simulink model "PI_VC_vs_UPI_CC_3ph_4w_v2023b"  (R2023b)
settings: Solver=FixedStepDiscrete  StartTime=0.0  StopTime=14  FixedStep=Ts_Power  MaxStep=1e-4  RelTol=1e-3
InitFcn:
  | run PI_VC_vs_UPI_CC_ini;
values from neighbouring files (symbols this model uses):
  C = 4e-6    (= 4e-06)    [PI_OL_vs_PI_CC_ini.m]    (also in PI_VC_vs_UPI_CC_ini.m)
  C_2 = 4e-6    (= 4e-06)    [PI_OL_vs_PI_CC_ini.m]    (also in PI_VC_vs_UPI_CC_ini.m)
  K_i_pll = 1.8/0.00251    (= 717.131474104)    [PI_OL_vs_PI_CC_ini.m]    (also in PI_VC_vs_UPI_CC_ini.m)
  K_p_pll = 1.8    [PI_OL_vs_PI_CC_ini.m]    (also in PI_VC_vs_UPI_CC_ini.m)
  Kp_i = 1*(L_t2 + L_s2)/tau_i    (= 2.5)    [PI_OL_vs_PI_CC_ini.m]    (also in PI_VC_vs_UPI_CC_ini.m)
  Kr_i = 2*(R_t2 + R_s2)/tau_i    (= 157.079632679)    [PI_OL_vs_PI_CC_ini.m]    (also in PI_VC_vs_UPI_CC_ini.m)
  L_line_12_13 = X_line_12_13/(2*pi*50)    (= 0.000798957814321)    [PI_OL_vs_PI_CC_ini.m]    (also in PI_VC_vs_UPI_CC_ini.m)
  L_line_13_14 = X_line_13_14/(2*pi*50)    (= 0.000200535228296)    [PI_OL_vs_PI_CC_ini.m]    (also in PI_VC_vs_UPI_CC_ini.m)
  L_n = L_t2 + L_s2    (= 0.0025)    [PI_OL_vs_PI_CC_ini.m]    (also in PI_VC_vs_UPI_CC_ini.m)
  L_s = 1.25e-3    (= 0.00125)    [PI_OL_vs_PI_CC_ini.m]    (also in PI_VC_vs_UPI_CC_ini.m)
  L_s2 = 1.25e-3    (= 0.00125)    [PI_OL_vs_PI_CC_ini.m]    (also in PI_VC_vs_UPI_CC_ini.m)
  L_t = 1.25e-3    (= 0.00125)    [PI_OL_vs_PI_CC_ini.m]    (also in PI_VC_vs_UPI_CC_ini.m)
  L_t2 = 1.25e-3    (= 0.00125)    [PI_OL_vs_PI_CC_ini.m]    (also in PI_VC_vs_UPI_CC_ini.m)
  omega = 2*pi*f    (= 314.159265359)    [PI_OL_vs_PI_CC_ini.m]    (also in PI_VC_vs_UPI_CC_ini.m)
  params_pi_cc = [S_b,U_b,K_p,T_p,K_q,T_q,X,R]    [PI_OL_vs_PI_CC_ini.m]    (also in PI_VC_vs_UPI_CC_ini.m)
  params_pi_vc = [S_b,U_b,K_p,T_p,K_q,T_q,Xv,Rv]    [PI_OL_vs_PI_CC_ini.m]    (also in PI_VC_vs_UPI_CC_ini.m)
  params_vc_cc = [R_t;L_t;R_s;L_s;K_pi;K_ii;C;K_pv;K_iv]    [PI_OL_vs_PI_CC_ini.m]    (also in PI_VC_vs_UPI_CC_ini.m)
  R_d = 10    [PI_OL_vs_PI_CC_ini.m]    (also in PI_VC_vs_UPI_CC_ini.m)
  R_d2 = 10    [PI_OL_vs_PI_CC_ini.m]    (also in PI_VC_vs_UPI_CC_ini.m)
  R_line_12_13 = (0.06)*Length    (= 0.24)    [PI_OL_vs_PI_CC_ini.m]    (also in PI_VC_vs_UPI_CC_ini.m)
  R_line_13_14 = (0.025)*Length    (= 0.1)    [PI_OL_vs_PI_CC_ini.m]    (also in PI_VC_vs_UPI_CC_ini.m)
  R_n = L_n*omega/10    (= 0.0785398163397)    [PI_OL_vs_PI_CC_ini.m]    (also in PI_VC_vs_UPI_CC_ini.m)
  R_s = L_s*omega/10    (= 0.0392699081699)    [PI_OL_vs_PI_CC_ini.m]    (also in PI_VC_vs_UPI_CC_ini.m)
  R_s2 = L_s*omega/10    (= 0.0392699081699)    [PI_OL_vs_PI_CC_ini.m]    (also in PI_VC_vs_UPI_CC_ini.m)
  R_t = L_t*omega/10    (= 0.0392699081699)    [PI_OL_vs_PI_CC_ini.m]    (also in PI_VC_vs_UPI_CC_ini.m)
  R_t2 = L_t*omega/10    (= 0.0392699081699)    [PI_OL_vs_PI_CC_ini.m]    (also in PI_VC_vs_UPI_CC_ini.m)
  S_b = 20e3    (= 20000)    [PI_OL_vs_PI_CC_ini.m]    (also in PI_VC_vs_UPI_CC_ini.m)
  Ts_Control = 50e-6    (= 5e-05)    [PI_OL_vs_PI_CC_ini.m]    (also in PI_VC_vs_UPI_CC_ini.m)
  Ts_Power = 50e-6    (= 5e-05)    [PI_OL_vs_PI_CC_ini.m]    (also in PI_VC_vs_UPI_CC_ini.m)
  v_dc = 800    [PI_OL_vs_PI_CC_ini.m]    (also in PI_VC_vs_UPI_CC_ini.m)
undefined symbols (not defined in the file or in its folder): DiscIntNeverNeededParam, omega_ref
libraries: spsFirstOrderFilterLib x32, spsUniversalBridgeLib x10, spsThreePhaseSeriesRLCBranchLib x9, spsPowerLib x6, spsThreePhaseVIMeasurementLib x6, eeGeneralControl x5, spsSeriesRLCLoadLib x5, spsRMSLib x4, spsSeriesRLCBranchLib x4, spsPower3phInstantaneousLib x3, spsThreePhaseBreakerLib x3, spsDCVoltageSourceLib x2
(part 1 of 3)
settings Model: Creator=Manuel  LastModifiedBy=iberi
settings SolverCC: AlgebraicLoopSolver=TrustRegion
settings DataIOCC: ReturnWorkspaceOutputs=off
settings DebuggingCC: UnconnectedInputMsg=warning  UnconnectedOutputMsg=warning  UnconnectedLineMsg=warning  ArithmeticOperatorsInVariantConditions=warning
settings ModelReferenceCC: EnableRefExpFcnMdlSchedulingChecks=on
settings SFSimCC: SimUseLocalCustomCode=off  CustomCodeUndefinedFunction=UseInterfaceOnly
settings RTWCC: RTWUseLocalCustomCode=off  DLArmComputeVersion=19.05

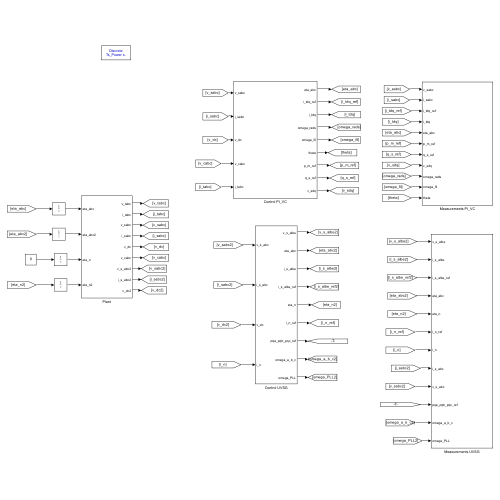
[thumbnail: Simulink's stored preview of the top-level diagram]
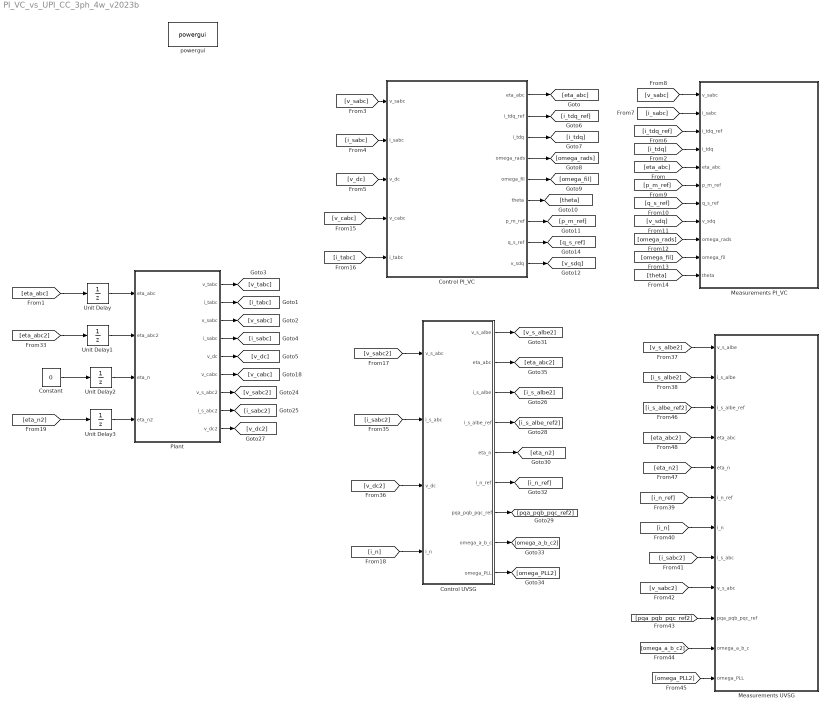
== system PI_VC_vs_UPI_CC_3ph_4w_v2023b ==
  Constant : Constant  Value=0
  Control PI_VC : Subsystem
  Control UVSG : Subsystem
  Measurements PI_VC : Subsystem
  Measurements UVSG : Subsystem
  Plant : Subsystem
  Unit Delay{,1..3} (4 alike) : UnitDelay  SampleTime=-1  HasFrameUpgradeWarning=on
  powergui : spspowerguiLib/powergui  Priority=1  SimulationMode=Discrete  SampleTime=Ts_Power  frequency=60  Iterations=50  frequencyindice=0  Pbase=100e6  ErrMax=1e-4  UnitsV=kV  UnitsW=MW  buscounter=0  FunctionMessages=off  echomessages=off  EnableUseOfTLC=off  CurrentSourceSwitches=off  DisableSnubberDevices=off  DisableRonSwitches=off  DisableVfSwitches=off  DisplayEquations=off  AutomaticDiscreteSolvers=off  SolverType=Tustin/Backward Euler (TBE)  Interpol=off  ExternalGateDelay=off  methode=off  Ts=100  x0status=blocks  SPID=on  SwTol=0  HookPort=off  NonlinearTolerance=1e-4  nMaxIteration=100  ContinueOnMaxIteration=off  RestoreLinks=warning  ResistiveCurrentMeasurement=off  Frange=[0:2:500]  Ylog=off  Xlog=on  ShowGrid=off  save=off  variable=ZData  structure=v_sabc  ZoomFFT=off  StartTime=4  cycles=5  DisplayStyle=2  fundamental=50  FreqAxis=off  MaxFrequency=10000  frequencyindicesteady=1  RmsSteady=1  display=off
  wires:
  [v_sabc] -> Control PI_VC/1(v_sabc)
  [i_sabc] -> Control PI_VC/2(i_sabc)
  [v_dc] -> Control PI_VC/3(v_dc)
  Control PI_VC/1(eta_abc) -> [eta_abc]
  Control PI_VC/2(i_tdq_ref) -> [i_tdq_ref]
  Control PI_VC/3(i_tdq) -> [i_tdq]
  Control PI_VC/4(omega_rads) -> [omega_rads]
  Control PI_VC/5(omega_fil) -> [omega_fil]
  Control PI_VC/6(theta) -> [theta]
  Control PI_VC/7(p_m_ref) -> [p_m_ref]
  Control PI_VC/8(q_s_ref) -> [q_s_ref]
  Control PI_VC/9(v_sdq) -> [v_sdq]
  [eta_abc] -> Measurements PI_VC/5(eta_abc)
  [i_tdq] -> Measurements PI_VC/4(i_tdq)
  [i_tdq_ref] -> Measurements PI_VC/3(i_tdq_ref)
  [i_sabc] -> Measurements PI_VC/2(i_sabc)
  [v_sabc] -> Measurements PI_VC/1(v_sabc)
  [p_m_ref] -> Measurements PI_VC/6(p_m_ref)
  [q_s_ref] -> Measurements PI_VC/7(q_s_ref)
  [v_sdq] -> Measurements PI_VC/8(v_sdq)
  [omega_rads] -> Measurements PI_VC/9(omega_rads)
  [omega_fil] -> Measurements PI_VC/10(omega_fil)
  [theta] -> Measurements PI_VC/11(theta)
  [v_cabc] -> Control PI_VC/4(v_cabc)
  [i_tabc] -> Control PI_VC/5(i_tabc)
  Plant/2(i_tabc) -> [i_tabc]
  Plant/6(v_cabc) -> [v_cabc]
  [eta_abc2] -> Unit Delay1/1
  [eta_abc] -> Unit Delay/1
  Plant/7(v_s_abc2) -> [v_sabc2]
  Plant/9(v_dc2) -> [v_dc2]
  Constant/1 -> Unit Delay2/1
  Unit Delay/1 -> Plant/1(eta_abc)
  Plant/5(v_dc) -> [v_dc]
  Unit Delay1/1 -> Plant/2(eta_abc2)
  Plant/8(i_s_abc2) -> [i_sabc2]
  Plant/3(v_sabc) -> [v_sabc]
  Plant/1(v_tabc) -> [v_tabc]
  Plant/4(i_sabc) -> [i_sabc]
  Unit Delay2/1 -> Plant/3(eta_n)
  [eta_n2] -> Unit Delay3/1
  Unit Delay3/1 -> Plant/4(eta_n2)
  Control UVSG/4(i_s_albe_ref) -> [i_s_albe_ref2]
  Control UVSG/5(eta_n) -> [eta_n2]
  [i_sabc2] -> Control UVSG/2(i_s_abc)
  [i_s_albe2] -> Measurements UVSG/2(i_s_albe)
  [v_s_albe2] -> Measurements UVSG/1(v_s_albe)
  [i_n] -> Measurements UVSG/7(i_n)
  [v_sabc2] -> Control UVSG/1(v_s_abc)
  [eta_abc2] -> Measurements UVSG/4(eta_abc)
  [i_s_albe_ref2] -> Measurements UVSG/3(i_s_albe_ref)
  [v_dc2] -> Control UVSG/3(v_dc)
  Control UVSG/9(omega_PLL) -> [omega_PLL2]
  Control UVSG/6(i_n_ref) -> [i_n_ref]
  [v_sabc2] -> Measurements UVSG/9(v_s_abc)
  [pqa_pqb_pqc_ref2] -> Measurements UVSG/10(pqa_pqb_pqc_ref)
  [omega_a_b_c2] -> Measurements UVSG/11(omega_a_b_c)
  Control UVSG/7(pqa_pqb_pqc_ref) -> [pqa_pqb_pqc_ref2]
  [i_sabc2] -> Measurements UVSG/8(i_s_abc)
  Control UVSG/8(omega_a_b_c) -> [omega_a_b_c2]
  [eta_n2] -> Measurements UVSG/5(eta_n)
  [omega_PLL2] -> Measurements UVSG/12(omega_PLL)
  [i_n] -> Control UVSG/4(i_n)
  [i_n_ref] -> Measurements UVSG/6(i_n_ref)
  Control UVSG/2(eta_abc) -> [eta_abc2]
  Control UVSG/3(i_s_albe) -> [i_s_albe2]
  Control UVSG/1(v_s_albe) -> [v_s_albe2]

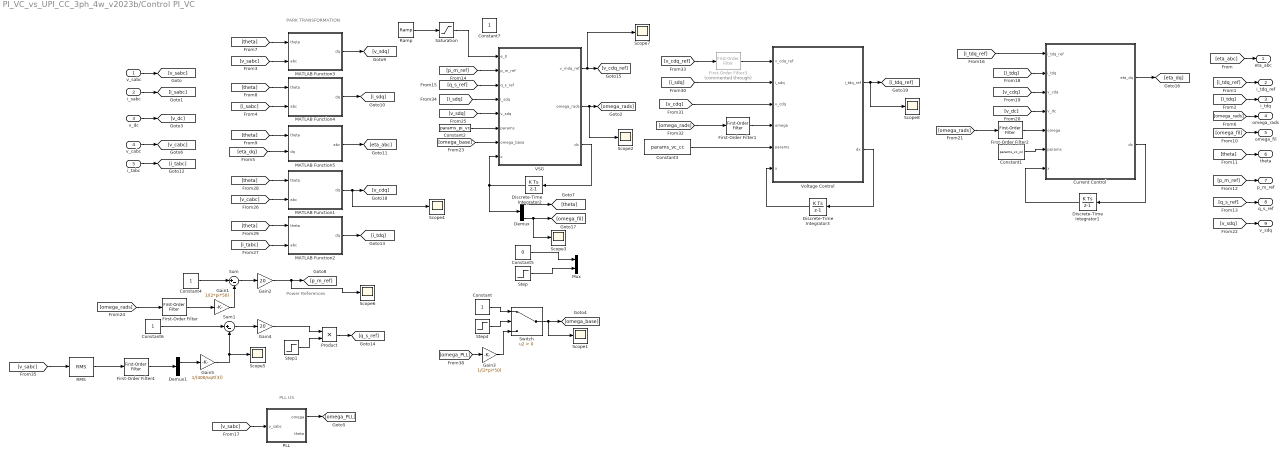
== system PI_VC_vs_UPI_CC_3ph_4w_v2023b/Control PI_VC ==
  note: PARK TRANSFORMATION
  note: Power References
  note: PLL US
  v_sabc : Inport
  i_sabc : Inport  Port=2
  v_dc : Inport  Port=3
  v_cabc : Inport  Port=4
  i_tabc : Inport  Port=5
  Constant{,4,6..7} (4 alike) : Constant
  Constant1 : Constant  Value=params_vc_cc
  Constant2 : Constant  Value=params_pi_vc
  Constant3 : Constant  Value=params_vc_cc
  Constant5 : Constant  Value=0
  Current Control : MATLAB Function  TreatAsAtomicUnit=on
  Demux : Demux
  Demux1 : Demux  Outputs=3
  Discrete-Time Integrator1 : DiscreteIntegrator  InitialCondition=[0;0]  SampleTime=Ts_Control  ICPrevOutput=DiscIntNeverNeededParam  ICPrevScaledInput=DiscIntNeverNeededParam
  Discrete-Time Integrator2 : DiscreteIntegrator  InitialCondition=[0;0;0;2*pi*50]  SampleTime=Ts_Control  ICPrevOutput=DiscIntNeverNeededParam  ICPrevScaledInput=DiscIntNeverNeededParam
  Discrete-Time Integrator3 : DiscreteIntegrator  InitialCondition=[0;0]  SampleTime=Ts_Control  ICPrevOutput=DiscIntNeverNeededParam  ICPrevScaledInput=DiscIntNeverNeededParam
  First-Order Filter{,1..2,4} (4 alike) : spsFirstOrderFilterLib/First-Order Filter  FilterType=Lowpass  Tc=10e-3  Ts=Ts_Control  Initialize=on  Vac_Init=[0, 0, 60]  Vdc_Init=0  PlotResponse=off  FreqRange="[0,  200,  1]"
  First-Order Filter3 : spsFirstOrderFilterLib/First-Order Filter  Commented=through  FilterType=Lowpass  Tc=2.4e-3  Ts=Ts_Control  Initialize=on  Vac_Init=[0, 0, 60]  Vdc_Init=0  PlotResponse=off  FreqRange="[0,  200,  1]"
  Gain1 : Gain  Gain=1/(2*pi*50)
  Gain2 : Gain  Gain=20
  Gain3 : Gain  Gain=1/(2*pi*50)
  Gain4 : Gain  Gain=20
  Gain5 : Gain  Gain=1/(400/sqrt(3))
  MATLAB Function1 : MATLAB Function  TreatAsAtomicUnit=on
  MATLAB Function2 : MATLAB Function  TreatAsAtomicUnit=on
  MATLAB Function3 : MATLAB Function  TreatAsAtomicUnit=on
  MATLAB Function4 : MATLAB Function  TreatAsAtomicUnit=on
  MATLAB Function5 : MATLAB Function  TreatAsAtomicUnit=on
  Mux : Mux  Inputs=2
  PLL : Subsystem
  Product : Product
  RMS : spsRMSLib/RMS  TrueRMS=on  Freq=50  RMSInit=230  Ts=Ts_Control
  Ramp : simulink/Sources/Ramp  slope=1  start=0  InitialOutput=0
  Saturation : Saturate  UpperLimit=1  LowerLimit=-1
  Scope{1..8} (8 alike) : Scope
  Step : Step  After=-325  SampleTime=0
  Step1 : Step  Time=0  SampleTime=0
  Step4 : Step  Time=0  SampleTime=0
  Sum : Sum  Inputs=|+-
  Sum1 : Sum  Inputs=|+-
  Switch : Switch  Criteria=u2 > Threshold  SaturateOnIntegerOverflow=off  InputSameDT=off
  VSG : MATLAB Function  TreatAsAtomicUnit=on
  Voltage Control : MATLAB Function  TreatAsAtomicUnit=on
  eta_abc : Outport  VectorParamsAs1DForOutWhenUnconnected=off
  i_tdq_ref : Outport  Port=2  VectorParamsAs1DForOutWhenUnconnected=off
  i_tdq : Outport  Port=3  VectorParamsAs1DForOutWhenUnconnected=off
  omega_rads : Outport  Port=4  VectorParamsAs1DForOutWhenUnconnected=off
  omega_fil : Outport  Port=5  VectorParamsAs1DForOutWhenUnconnected=off
  theta : Outport  Port=6  VectorParamsAs1DForOutWhenUnconnected=off
  p_m_ref : Outport  Port=7  VectorParamsAs1DForOutWhenUnconnected=off
  q_s_ref : Outport  Port=8  VectorParamsAs1DForOutWhenUnconnected=off
  v_sdq : Outport  Port=9  VectorParamsAs1DForOutWhenUnconnected=off
  wires:
  [theta] -> MATLAB Function4/1(theta)
  MATLAB Function5/1(abc) -> [eta_abc]
  [i_sabc] -> MATLAB Function4/2(abc)
  [eta_dq] -> MATLAB Function5/2(dq)
  Gain2/1 -> Scope6/1, [p_m_ref]
  MATLAB Function3/1(dq) -> [v_sdq]
  MATLAB Function4/1(dq) -> [i_sdq]
  [theta] -> MATLAB Function5/1(theta)
  [theta] -> MATLAB Function3/1(theta)
  [v_sabc] -> MATLAB Function3/2(abc)
  Discrete-Time Integrator2/1 -> Demux/1, VSG/8(x)
  Demux/4 -> Scope3/1, [omega_fil]
  Demux/1 -> [theta]
  [v_dc] -> Current Control/4(v_dc)
  Constant2/1 -> VSG/6(params)
  [p_m_ref] -> VSG/2(p_m_ref)
  Constant1/1 -> Current Control/6(params)
  Current Control/1(eta_dq) -> [eta_dq]
  [omega_rads] -> First-Order Filter2/1
  Current Control/2(dx) -> Discrete-Time Integrator1/1
  [q_s_ref] -> VSG/3(q_s_ref)
  Discrete-Time Integrator1/1 -> Current Control/7(x)
  VSG/3(dx) -> Discrete-Time Integrator2/1
  [v_cdq] -> Current Control/3(v_cdq)
  [i_tdq] -> Current Control/2(i_tdq)
  v_sabc/1 -> [v_sabc]
  i_sabc/1 -> [i_sabc]
  VSG/2(omega_rads) -> Scope2/1, [omega_rads]
  v_dc/1 -> [v_dc]
  [eta_abc] -> eta_abc/1
  [i_tdq_ref] -> i_tdq_ref/1
  [i_tdq] -> i_tdq/1
  [omega_rads] -> omega_rads/1
  [omega_fil] -> omega_fil/1
  [theta] -> theta/1
  [p_m_ref] -> p_m_ref/1
  [q_s_ref] -> q_s_ref/1
  [v_sabc] -> PLL/1(v_sabc)
  [v_sdq] -> v_sdq/1
  Switch/1 -> Scope1/1, [omega_base]
  Constant/1 -> Switch/1
  Gain3/1 -> Switch/3
  [omega_PLL] -> Gain3/1
  Step4/1 -> Switch/2
  PLL/1(omega) -> [omega_PLL]
  [omega_base] -> VSG/7(omega_base)
  i_tabc/1 -> [i_tabc]
  v_cabc/1 -> [v_cabc]
  [v_cabc] -> MATLAB Function1/2(abc)
  [theta] -> MATLAB Function1/1(theta)
  MATLAB Function2/1(dq) -> [i_tdq]
  MATLAB Function1/1(dq) -> Scope4/1, [v_cdq]
  [i_tabc] -> MATLAB Function2/2(abc)
  [theta] -> MATLAB Function2/1(theta)
  Voltage Control/2(dx) -> Discrete-Time Integrator3/1
  [i_sdq] -> Voltage Control/2(i_sdq)
  [v_cdq] -> Voltage Control/3(v_cdq)
  [omega_rads] -> First-Order Filter1/1
  Constant3/1 -> Voltage Control/5(params)
  Discrete-Time Integrator3/1 -> Voltage Control/6(x)
  Voltage Control/1(i_tdq_ref) -> Scope8/1, [i_tdq_ref]
  [v_cdq_ref] -> First-Order Filter3/1
  [i_sdq] -> VSG/4(i_sdq)
  [v_sdq] -> VSG/5(v_sdq)
  Constant5/1 -> Mux/1
  Step/1 -> Mux/2
  [omega_rads] -> First-Order Filter/1
  Gain1/1 -> Sum/2
  Sum/1 -> Gain2/1
  Sum1/1 -> Gain4/1
  VSG/1(v_mdq_ref) -> Scope7/1, [v_cdq_ref]
  [v_sabc] -> RMS/1
  RMS/1 -> First-Order Filter4/1
  Demux1/1 -> Gain5/1
  Gain5/1 -> Scope5/1, Sum1/2
  Constant4/1 -> Sum/1
  Ramp/1 -> Saturation/1
  Constant6/1 -> Sum1/1
  Product/1 -> [q_s_ref]
  Gain4/1 -> Product/1
  Step1/1 -> Product/2
  First-Order Filter/1 -> Gain1/1
  [i_tdq_ref] -> Current Control/1(i_tdq_ref)
  First-Order Filter1/1 -> Voltage Control/4(omega)
  First-Order Filter2/1 -> Current Control/5(omega)
  First-Order Filter3/1 -> Voltage Control/1(v_cdq_ref)
  First-Order Filter4/1 -> Demux1/1
  Saturation/1 -> VSG/1(e_0)

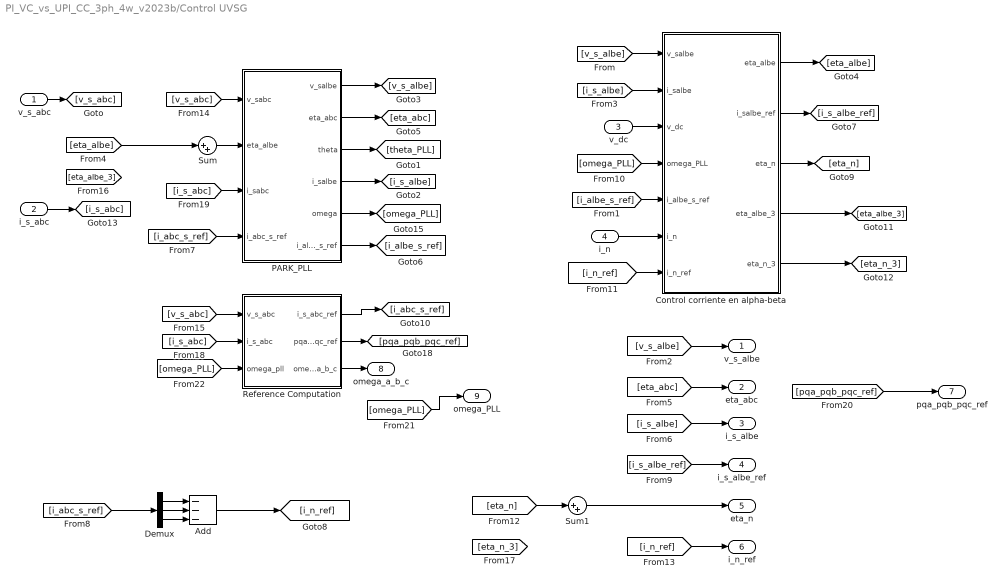
== system PI_VC_vs_UPI_CC_3ph_4w_v2023b/Control UVSG ==
  v_s_abc : Inport
  i_s_abc : Inport  Port=2
  v_dc : Inport  Port=3
  i_n : Inport  Port=4
  Add : Sum  Inputs=---
  Control corriente en alpha-beta : Subsystem
  Demux : Demux  Outputs=3
  PARK_PLL : Subsystem
  Reference Computation : Subsystem
  Sum : Sum  Inputs=|++
  Sum1 : Sum  Inputs=|++
  v_s_albe : Outport  VectorParamsAs1DForOutWhenUnconnected=off
  eta_abc : Outport  Port=2  VectorParamsAs1DForOutWhenUnconnected=off
  i_s_albe : Outport  Port=3  VectorParamsAs1DForOutWhenUnconnected=off
  i_s_albe_ref : Outport  Port=4  VectorParamsAs1DForOutWhenUnconnected=off
  eta_n : Outport  Port=5  VectorParamsAs1DForOutWhenUnconnected=off
  i_n_ref : Outport  Port=6  VectorParamsAs1DForOutWhenUnconnected=off
  pqa_pqb_pqc_ref : Outport  Port=7  VectorParamsAs1DForOutWhenUnconnected=off
  omega_a_b_c : Outport  Port=8  VectorParamsAs1DForOutWhenUnconnected=off
  omega_PLL : Outport  Port=9  VectorParamsAs1DForOutWhenUnconnected=off
  wires:
  Control corriente en alpha-beta/1(eta_albe) -> [eta_albe]
  [v_s_albe] -> Control corriente en alpha-beta/1(v_salbe)
  [i_s_albe] -> Control corriente en alpha-beta/2("i_salbe  ")
  [v_s_albe] -> v_s_albe/1
  [i_s_albe] -> i_s_albe/1
  [omega_PLL] -> Control corriente en alpha-beta/4(omega_PLL)
  Control corriente en alpha-beta/2(i_salbe_ref) -> [i_s_albe_ref]
  [i_s_albe_ref] -> i_s_albe_ref/1
  PARK_PLL/1(v_salbe) -> [v_s_albe]
  PARK_PLL/4(i_salbe) -> [i_s_albe]
  PARK_PLL/2(eta_abc) -> [eta_abc]
  PARK_PLL/5(omega) -> [omega_PLL]
  PARK_PLL/3(theta) -> [theta_PLL]
  v_dc/1 -> Control corriente en alpha-beta/3(v_dc)
  [i_albe_s_ref] -> Control corriente en alpha-beta/5(i_albe_s_ref)
  [i_abc_s_ref] -> PARK_PLL/4(i_abc_s_ref)
  PARK_PLL/6(i_albe_s_ref) -> [i_albe_s_ref]
  i_n/1 -> Control corriente en alpha-beta/6(i_n)
  Demux/2 -> Add/2
  Demux/3 -> Add/3
  [i_abc_s_ref] -> Demux/1
  Demux/1 -> Add/1
  Add/1 -> [i_n_ref]
  [i_n_ref] -> Control corriente en alpha-beta/7(i_n_ref)
  Control corriente en alpha-beta/3(eta_n) -> [eta_n]
  [i_n_ref] -> i_n_ref/1
  v_s_abc/1 -> [v_s_abc]
  [v_s_abc] -> PARK_PLL/1(v_sabc)
  [v_s_abc] -> Reference Computation/1(v_s_abc)
  Reference Computation/1(i_s_abc_ref) -> [i_abc_s_ref]
  Control corriente en alpha-beta/4(eta_albe_3) -> [eta_albe_3]
  Control corriente en alpha-beta/5(eta_n_3) -> [eta_n_3]
  [eta_abc] -> eta_abc/1
  [eta_n] -> Sum1/1
  Sum1/1 -> eta_n/1
  Sum/1 -> PARK_PLL/2(eta_albe)
  [eta_albe] -> Sum/1
  Reference Computation/2(pqa_pqb_pqc_ref) -> [pqa_pqb_pqc_ref]
  [i_s_abc] -> Reference Computation/2(i_s_abc)
  i_s_abc/1 -> [i_s_abc]
  [i_s_abc] -> PARK_PLL/3(i_sabc)
  [pqa_pqb_pqc_ref] -> pqa_pqb_pqc_ref/1
  Reference Computation/3(omega_a_b_c) -> omega_a_b_c/1
  [omega_PLL] -> omega_PLL/1
  [omega_PLL] -> Reference Computation/3(omega_pll)

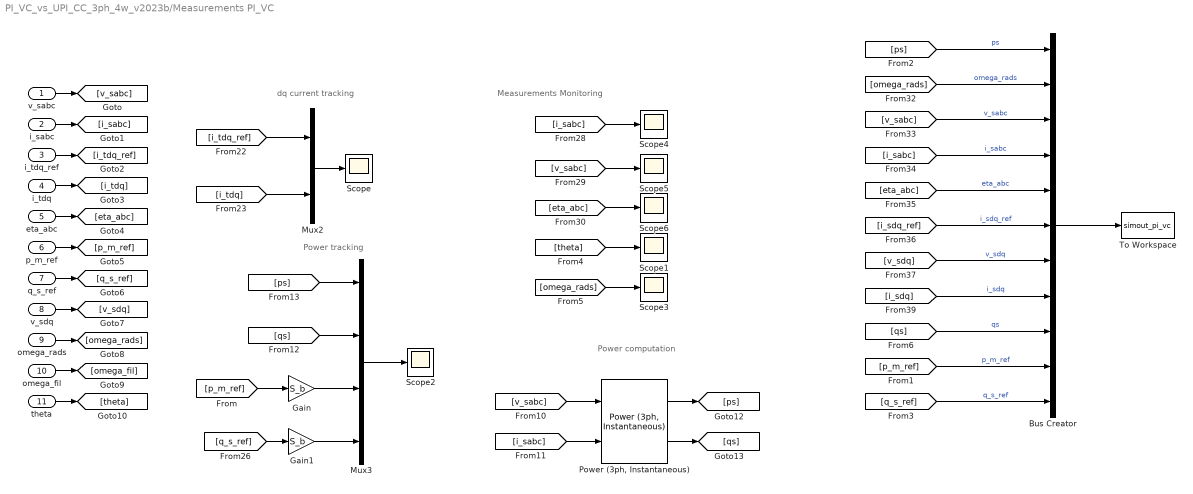
== system PI_VC_vs_UPI_CC_3ph_4w_v2023b/Measurements PI_VC ==
  note: Power computation
  note: dq current tracking
  note: Measurements Monitoring
  note: Power tracking
  v_sabc : Inport
  i_sabc : Inport  Port=2
  i_tdq_ref : Inport  Port=3
  i_tdq : Inport  Port=4
  eta_abc : Inport  Port=5
  p_m_ref : Inport  Port=6
  q_s_ref : Inport  Port=7
  v_sdq : Inport  Port=8
  omega_rads : Inport  Port=9
  omega_fil : Inport  Port=10
  theta : Inport  Port=11
  Bus Creator : BusCreator  Inputs=11
  Gain : Gain  Gain=S_b
  Gain1 : Gain  Gain=S_b
  Mux2 : Mux  Inputs=2
  Mux3 : Mux
  "Power (3ph, Instantaneous)" : spsPower3phInstantaneousLib/Power (3ph, Instantaneous)
  Scope{,1..6} (7 alike) : Scope
  To Workspace : ToWorkspace  VariableName=simout_pi_vc  SaveFormat=Timeseries  SampleTime=-1
  wires:
  [v_sdq] -> Bus Creator/7  "v_sdq"
  [i_tdq] -> Mux2/2
  [v_sabc] -> "Power (3ph, Instantaneous)"/1
  Mux2/1 -> Scope/1
  Gain1/1 -> Mux3/4
  Bus Creator/1 -> To Workspace/1
  [qs] -> Mux3/2
  [eta_abc] -> Scope6/1
  [omega_rads] -> Bus Creator/2  "omega_rads"
  [i_sdq] -> Bus Creator/8  "i_sdq"
  [i_tdq_ref] -> Mux2/1
  [p_m_ref] -> Gain/1
  [v_sabc] -> Bus Creator/3  "v_sabc"
  [ps] -> Bus Creator/1  "ps"
  [v_sabc] -> Scope5/1
  [i_sabc] -> "Power (3ph, Instantaneous)"/2
  "Power (3ph, Instantaneous)"/1 -> [ps]
  [i_sabc] -> Scope4/1
  "Power (3ph, Instantaneous)"/2 -> [qs]
  [q_s_ref] -> Gain1/1
  [eta_abc] -> Bus Creator/5  "eta_abc"
  [ps] -> Mux3/1
  [qs] -> Bus Creator/9  "qs"
  Gain/1 -> Mux3/3
  [i_sabc] -> Bus Creator/4  "i_sabc"
  Mux3/1 -> Scope2/1
  [i_sdq_ref] -> Bus Creator/6  "i_sdq_ref"
  v_sabc/1 -> [v_sabc]
  i_sabc/1 -> [i_sabc]
  i_tdq_ref/1 -> [i_tdq_ref]
  i_tdq/1 -> [i_tdq]
  eta_abc/1 -> [eta_abc]
  p_m_ref/1 -> [p_m_ref]
  q_s_ref/1 -> [q_s_ref]
  v_sdq/1 -> [v_sdq]
  omega_rads/1 -> [omega_rads]
  omega_fil/1 -> [omega_fil]
  [p_m_ref] -> Bus Creator/10  "p_m_ref"
  [q_s_ref] -> Bus Creator/11  "q_s_ref"
  theta/1 -> [theta]
  [theta] -> Scope1/1
  [omega_rads] -> Scope3/1

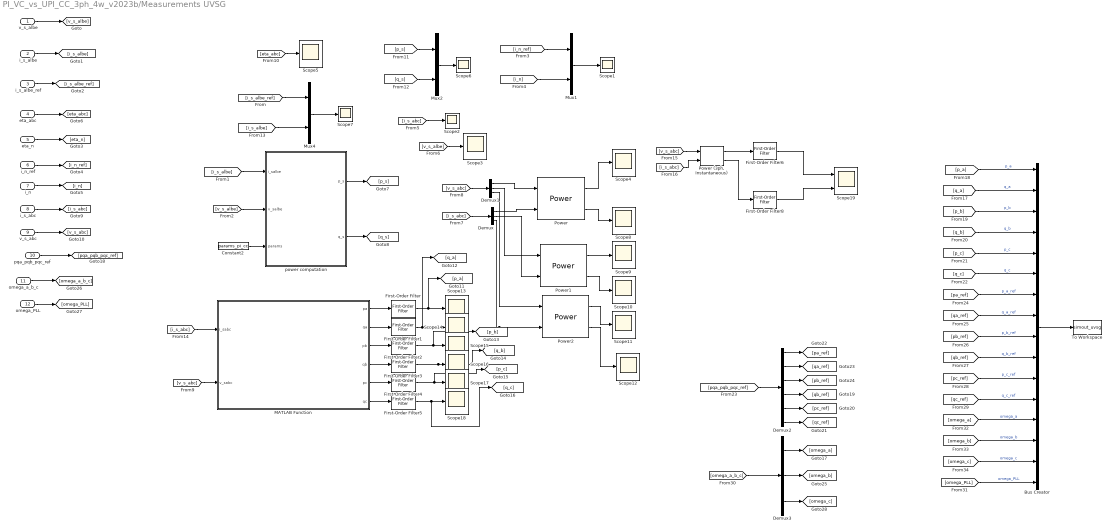
== system PI_VC_vs_UPI_CC_3ph_4w_v2023b/Measurements UVSG ==
  v_s_albe : Inport
  i_s_albe : Inport  Port=2
  i_s_albe_ref : Inport  Port=3
  eta_abc : Inport  Port=4
  eta_n : Inport  Port=5
  i_n_ref : Inport  Port=6
  i_n : Inport  Port=7
  i_s_abc : Inport  Port=8
  v_s_abc : Inport  Port=9
  pqa_pqb_pqc_ref : Inport  Port=10
  omega_a_b_c : Inport  Port=11
  omega_PLL : Inport  Port=12
  Bus Creator : BusCreator  Inputs=16
  Constant2 : Constant  Value=params_pi_cc
  Demux : Demux  Outputs=3
  Demux1 : Demux  Outputs=3
  Demux2 : Demux  Outputs=6
  Demux3 : Demux  Outputs=3
  First-Order Filter{,1..6,8} (8 alike) : spsFirstOrderFilterLib/First-Order Filter  FilterType=Lowpass  Tc=0.1  Ts=Ts_Control  Initialize=on  Vac_Init=[0, 0, 60]  Vdc_Init=0  PlotResponse=off  FreqRange="[0,  200,  1]"
  MATLAB Function : MATLAB Function  TreatAsAtomicUnit=on
  Mux1 : Mux  Inputs=2
  Mux2 : Mux  Inputs=2
  Mux4 : Mux  Inputs=2
  Power : spsPowerLib/Power  Freq=50  Vinit=[1, 0]  Iinit=[1, 0]  Ts=Ts_Control
  "Power (3ph, Instantaneous)" : spsPower3phInstantaneousLib/Power (3ph, Instantaneous)
  Power1 : spsPowerLib/Power  Freq=50  Vinit=[1, 0]  Iinit=[1, 0]  Ts=Ts_Control
  Power2 : spsPowerLib/Power  Freq=50  Vinit=[1, 0]  Iinit=[1, 0]  Ts=Ts_Control
  Scope{1..18} (18 alike) : Scope
  Scope19 : Scope  NumInputPorts=2
  To Workspace : ToWorkspace  VariableName=simout_uvsg  SaveFormat=Timeseries  SampleTime=-1
  power computation : MATLAB Function  TreatAsAtomicUnit=on
  wires:
  [eta_abc] -> Scope5/1
  [v_s_albe] -> Scope3/1
  Mux2/1 -> Scope6/1
  [p_s] -> Mux2/1
  Mux4/1 -> Scope7/1
  [i_s_albe_ref] -> Mux4/1
  [i_s_albe] -> Mux4/2
  [q_s] -> Mux2/2
  v_s_albe/1 -> [v_s_albe]
  i_s_albe/1 -> [i_s_albe]
  i_s_albe_ref/1 -> [i_s_albe_ref]
  eta_abc/1 -> [eta_abc]
  Constant2/1 -> power computation/3(params)
  power computation/2(q_s) -> [q_s]
  power computation/1(p_s) -> [p_s]
  [v_s_albe] -> power computation/2(v_salbe)
  [i_s_albe] -> power computation/1(i_salbe)
  eta_n/1 -> [eta_n]
  i_n_ref/1 -> [i_n_ref]
  i_n/1 -> [i_n]
  [i_n] -> Mux1/2
  [i_n_ref] -> Mux1/1
  Mux1/1 -> Scope1/1
  i_s_abc/1 -> [i_s_abc]
  [i_s_abc] -> Scope2/1
  v_s_abc/1 -> [v_s_abc]
  [i_s_abc] -> Demux/1
  [v_s_abc] -> Demux1/1
  Power/1 -> Scope4/1
  Power/2 -> Scope8/1
  Demux1/1 -> Power/1
  Demux/1 -> Power/2
  Demux1/2 -> Power1/1
  Demux/2 -> Power1/2
  Demux1/3 -> Power2/1
  Demux/3 -> Power2/2
  Power1/1 -> Scope9/1
  Power1/2 -> Scope10/1
  Power2/1 -> Scope11/1
  Power2/2 -> Scope12/1
  [v_s_abc] -> MATLAB Function/2(v_sabc)
  [i_s_abc] -> MATLAB Function/1(i_sabc)
  MATLAB Function/1(pa) -> First-Order Filter/1
  MATLAB Function/2(qa) -> First-Order Filter1/1
  MATLAB Function/3(pb) -> First-Order Filter2/1
  MATLAB Function/4(qb) -> First-Order Filter3/1
  MATLAB Function/5(pc) -> First-Order Filter4/1
  MATLAB Function/6(qc) -> First-Order Filter5/1
  First-Order Filter/1 -> [p_a], Scope13/1
  First-Order Filter1/1 -> [q_a], Scope14/1
  First-Order Filter2/1 -> [p_b], Scope15/1
  First-Order Filter3/1 -> [q_b], Scope16/1
  First-Order Filter4/1 -> [p_c], Scope17/1
  First-Order Filter5/1 -> [q_c], Scope18/1
  [v_s_abc] -> "Power (3ph, Instantaneous)"/1
  [i_s_abc] -> "Power (3ph, Instantaneous)"/2
  "Power (3ph, Instantaneous)"/1 -> First-Order Filter6/1
  First-Order Filter6/1 -> Scope19/1
  First-Order Filter8/1 -> Scope19/2
  "Power (3ph, Instantaneous)"/2 -> First-Order Filter8/1
  Bus Creator/1 -> To Workspace/1
  ? -> ?
  [p_a] -> Bus Creator/1  "p_a"
  [q_a] -> Bus Creator/2  "q_a"
  Demux2/5 -> [pc_ref]
  Demux2/4 -> [qb_ref]
  Demux2/6 -> [qc_ref]
  [pqa_pqb_pqc_ref] -> Demux2/1
  Demux2/3 -> [pb_ref]
  Demux2/2 -> [qa_ref]
  Demux2/1 -> [pa_ref]
  pqa_pqb_pqc_ref/1 -> [pqa_pqb_pqc_ref]
  omega_a_b_c/1 -> [omega_a_b_c]
  omega_PLL/1 -> [omega_PLL]
  [omega_a_b_c] -> Demux3/1
  Demux3/2 -> [omega_b]
  Demux3/3 -> [omega_c]
  Demux3/1 -> [omega_a]
  [q_b] -> Bus Creator/4  "q_b"
  [p_b] -> Bus Creator/3  "p_b"
  [p_c] -> Bus Creator/5  "p_c"
  [omega_PLL] -> Bus Creator/16  "omega_PLL"
  [q_c] -> Bus Creator/6  "q_c"
  [pa_ref] -> Bus Creator/7  "p_a_ref"
  [omega_c] -> Bus Creator/15  "omega_c"
  [qa_ref] -> Bus Creator/8  "q_a_ref"
  [omega_b] -> Bus Creator/14  "omega_b"
  [pb_ref] -> Bus Creator/9  "p_b_ref"
  [omega_a] -> Bus Creator/13  "omega_a"
  [qb_ref] -> Bus Creator/10  "q_b_ref"
  [qc_ref] -> Bus Creator/12  "q_c_ref"
  [pc_ref] -> Bus Creator/11  "p_c_ref"

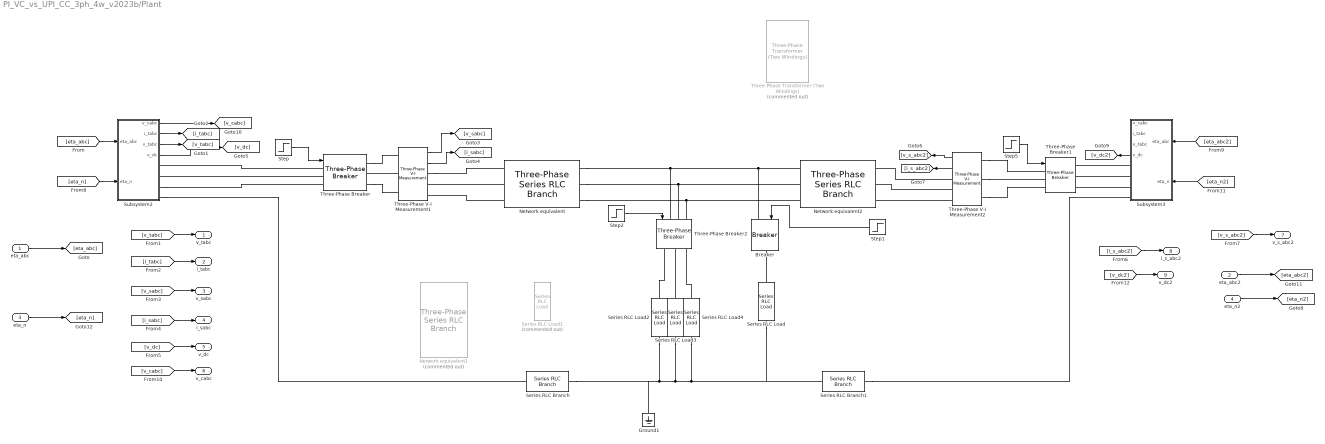
== system PI_VC_vs_UPI_CC_3ph_4w_v2023b/Plant ==
  eta_abc : Inport
  eta_abc2 : Inport  Port=2
  eta_n : Inport  Port=3
  eta_n2 : Inport  Port=4
  Breaker : spsBreakerLib/Breaker  InitialState=0  SwitchingTimes="[1/60  5/60]"  External=on  BreakerResistance=0.01  SnubberResistance=1e6  SnubberCapacitance=inf  Measurements=None  MoreParameters=on  NoBreakLoop=off
  Ground1 : spsGroundLib/Ground  LConnTagsString=a
  Network equivalent : spsThreePhaseSeriesRLCBranchLib/Three-Phase Series RLC Branch  LConnTagsString=A|B|C  RConnTagsString=A|B|C  BranchType=RL  Resistance=R_line_12_13  Inductance=L_line_12_13  Capacitance=1e-6  Measurements=None
  Network equivalent1 : spsThreePhaseSeriesRLCBranchLib/Three-Phase Series RLC Branch  Commented=on  LConnTagsString=A|B|C  RConnTagsString=A|B|C  BranchType=RL  Resistance=25  Inductance=12/(2*pi*50)  Capacitance=1e-6  Measurements=None
  Network equivalent2 : spsThreePhaseSeriesRLCBranchLib/Three-Phase Series RLC Branch  LConnTagsString=A|B|C  RConnTagsString=A|B|C  BranchType=RL  Resistance=R_line_13_14  Inductance=L_line_13_14  Capacitance=1e-6  Measurements=None
  Series RLC Branch : spsSeriesRLCBranchLib/Series RLC Branch  LConnTagsString=__new0  RConnTagsString=__new0  BranchType=RL  Resistance=R_line_12_13  Inductance=L_line_12_13  SetiL0=off  InitialCurrent=0  Capacitance=1e-6  Setx0=off  InitialVoltage=0  Measurements=None
  Series RLC Branch1 : spsSeriesRLCBranchLib/Series RLC Branch  LConnTagsString=__new0  RConnTagsString=__new0  BranchType=RL  Resistance=R_line_13_14  Inductance=L_line_13_14  SetiL0=off  InitialCurrent=0  Capacitance=1e-6  Setx0=off  InitialVoltage=0  Measurements=None
  Series RLC Load : spsSeriesRLCLoadLib/Series RLC Load  LConnTagsString=a  RConnTagsString=__new0  NominalVoltage=230  NominalFrequency=50  ActivePower=1e3  InductivePower=1e3  CapacitivePower=0  Setx0=off  InitialVoltage=0  SetiL0=off  InitialCurrent=0  Measurements=None  LoadType=constant Z
  Series RLC Load1 : spsSeriesRLCLoadLib/Series RLC Load  Commented=on  LConnTagsString=a  RConnTagsString=__new0  NominalVoltage=230  NominalFrequency=50  ActivePower=1e3  InductivePower=1e3  CapacitivePower=0  Setx0=off  InitialVoltage=0  SetiL0=off  InitialCurrent=0  Measurements=None  LoadType=constant Z
  Series RLC Load2 : spsSeriesRLCLoadLib/Series RLC Load  LConnTagsString=a  RConnTagsString=__new0  NominalVoltage=230  NominalFrequency=50  ActivePower=2e3  InductivePower=500  CapacitivePower=0  Setx0=off  InitialVoltage=0  SetiL0=off  InitialCurrent=0  Measurements=None  LoadType=constant Z
  Series RLC Load3 : spsSeriesRLCLoadLib/Series RLC Load  LConnTagsString=a  RConnTagsString=__new0  NominalVoltage=230  NominalFrequency=50  ActivePower=2e3  InductivePower=500  CapacitivePower=0  Setx0=off  InitialVoltage=0  SetiL0=off  InitialCurrent=0  Measurements=None  LoadType=constant Z
  Series RLC Load4 : spsSeriesRLCLoadLib/Series RLC Load  LConnTagsString=a  RConnTagsString=__new0  NominalVoltage=230  NominalFrequency=50  ActivePower=2e3  InductivePower=500  CapacitivePower=0  Setx0=off  InitialVoltage=0  SetiL0=off  InitialCurrent=0  Measurements=None  LoadType=constant Z
  Step : Step  Time=0  SampleTime=0
  Step1 : Step  Time=9  SampleTime=0
  Step2 : Step  Time=3  SampleTime=0
  Step5 : Step  SampleTime=0
  Subsystem2 : Subsystem
  Subsystem3 : Subsystem
  Three-Phase Transformer (Two Windings) : spsThreePhaseTransformerTwoWindingsLib/Three-Phase Transformer (Two Windings)  Commented=on  Winding1Connection=Yn  Winding2Connection=Yn  CoreType=Three single-phase transformers  SetSaturation=off  Hysteresis=off  DataFile='hysteresis'  SetInitialFlux=off  Measurements=None  UNITS=pu  NominalPower=[ 125e3 , 50 ]  Winding1=[ 400 , 0.002 , 0.08 ]  Winding2=[ 400 , 0.002 , 0.08 ]  Rm=500  Lm=500  L0=0.5  Saturation=[ 0,0 ; 0.0024,1.2 ; 1.0,1.52 ]  InitialFluxes=[ 0.8 , -0.8 , 0.7 ]  BreakLoop=off  DiscreteSolver=Trapezoidal iterative  DataType=off  TransfoNumber=1
  Three-Phase V-I Measurement1 : spsThreePhaseVIMeasurementLib/Three-Phase V-I Measurement  VoltageMeasurement=phase-to-ground  SetLabelV=off  LabelV=Vabc  Vpu=off  VpuLL=off  CurrentMeasurement=yes  SetLabelI=off  LabelI=Iabc  Ipu=off  Pbase=100e6  Vbase=500e3  OutputType=Complex  PhasorSimulation=off  PSBequivalent=0
  Three-Phase V-I Measurement2 : spsThreePhaseVIMeasurementLib/Three-Phase V-I Measurement  VoltageMeasurement=phase-to-ground  SetLabelV=off  LabelV=Vabc  Vpu=off  VpuLL=off  CurrentMeasurement=yes  SetLabelI=off  LabelI=Iabc  Ipu=off  Pbase=100e6  Vbase=500e3  OutputType=Complex  PhasorSimulation=off  PSBequivalent=0
  Three-Phase Breaker : spsThreePhaseBreakerLib/Three-Phase Breaker  InitialState=open  SwitchA=on  SwitchB=on  SwitchC=on  SwitchTimes="[1/60  5/60]"  External=on  BreakerResistance=0.01  SnubberResistance=1e6  SnubberCapacitance=inf  Measurements=None
  Three-Phase Breaker1 : spsThreePhaseBreakerLib/Three-Phase Breaker  InitialState=open  SwitchA=on  SwitchB=on  SwitchC=on  SwitchTimes="[1/60  5/60]"  External=on  BreakerResistance=0.01  SnubberResistance=1e6  SnubberCapacitance=inf  Measurements=None
  Three-Phase Breaker2 : spsThreePhaseBreakerLib/Three-Phase Breaker  InitialState=open  SwitchA=on  SwitchB=on  SwitchC=on  SwitchTimes="[1/60  5/60]"  External=on  BreakerResistance=0.01  SnubberResistance=1e6  SnubberCapacitance=inf  Measurements=None
  v_tabc : Outport  VectorParamsAs1DForOutWhenUnconnected=off
  i_tabc : Outport  Port=2  VectorParamsAs1DForOutWhenUnconnected=off
  v_sabc : Outport  Port=3  VectorParamsAs1DForOutWhenUnconnected=off
  i_sabc : Outport  Port=4  VectorParamsAs1DForOutWhenUnconnected=off
  v_dc : Outport  Port=5  VectorParamsAs1DForOutWhenUnconnected=off
  v_cabc : Outport  Port=6  VectorParamsAs1DForOutWhenUnconnected=off
  v_s_abc2 : Outport  Port=7  VectorParamsAs1DForOutWhenUnconnected=off
  i_s_abc2 : Outport  Port=8  VectorParamsAs1DForOutWhenUnconnected=off
  v_dc2 : Outport  Port=9  VectorParamsAs1DForOutWhenUnconnected=off
  wires:
  Three-Phase V-I Measurement1/1 -> [v_sabc]
  Three-Phase V-I Measurement1/2 -> [i_sabc]
  [v_tabc] -> v_tabc/1
  [i_tabc] -> i_tabc/1
  [v_sabc] -> v_sabc/1
  [i_sabc] -> i_sabc/1
  eta_abc/1 -> [eta_abc]
  [v_dc] -> v_dc/1
  [v_cabc] -> v_cabc/1
  Step/1 -> Three-Phase Breaker/1
  Three-Phase V-I Measurement2/2 -> [i_s_abc2]
  Three-Phase V-I Measurement2/1 -> [v_s_abc2]
  Step5/1 -> Three-Phase Breaker1/1
  [i_s_abc2] -> i_s_abc2/1
  [v_s_abc2] -> v_s_abc2/1
  eta_abc2/1 -> [eta_abc2]
  eta_n/1 -> [eta_n]
  [v_dc2] -> v_dc2/1
  [eta_abc] -> Subsystem2/1(eta_abc)
  Subsystem2/1(v_cabc) -> [v_cabc]
  Subsystem2/2(i_tabc) -> [i_tabc]
  Subsystem2/3(v_tabc) -> [v_tabc]
  Subsystem2/4(v_dc) -> [v_dc]
  [eta_abc2] -> Subsystem3/1(eta_abc)
  Subsystem3/4(v_dc) -> [v_dc2]
  [eta_n] -> Subsystem2/2(eta_n)
  eta_n2/1 -> [eta_n2]
  [eta_n2] -> Subsystem3/2(eta_n)
  Step1/1 -> Breaker/1
  Step2/1 -> Three-Phase Breaker2/1
  connections:
  Three-Phase Breaker/RConn3 -- Three-Phase V-I Measurement1/LConn3
  Three-Phase V-I Measurement1/LConn2 -- Three-Phase Breaker/RConn2
  Three-Phase Breaker/RConn1 -- Three-Phase V-I Measurement1/LConn1
  Series RLC Load/RConn1 -- Series RLC Branch1/LConn1 -- Series RLC Load4/RConn1 -- Series RLC Load3/RConn1 -- Series RLC Load2/RConn1 -- Series RLC Branch/RConn1 -- Ground1/LConn1
  Subsystem3/RConn2 -- Three-Phase Breaker1/RConn2
  Subsystem3/RConn3 -- Three-Phase Breaker1/RConn3
  Subsystem3/RConn1 -- Three-Phase Breaker1/RConn1
  Three-Phase V-I Measurement2/LConn2 -- Three-Phase Breaker1/LConn2
  Three-Phase V-I Measurement2/LConn3 -- Three-Phase Breaker1/LConn3
  Three-Phase V-I Measurement2/LConn1 -- Three-Phase Breaker1/LConn1
  Three-Phase V-I Measurement2/RConn2 -- Network equivalent2/RConn2
  Three-Phase V-I Measurement2/RConn3 -- Network equivalent2/RConn3
  Three-Phase V-I Measurement2/RConn1 -- Network equivalent2/RConn1
  Three-Phase Breaker/LConn1 -- Subsystem2/RConn1
  Three-Phase Breaker/LConn2 -- Subsystem2/RConn2
  Subsystem2/RConn3 -- Three-Phase Breaker/LConn3
  Network equivalent/LConn2 -- Three-Phase V-I Measurement1/RConn2
  Network equivalent/LConn3 -- Three-Phase V-I Measurement1/RConn3
  Three-Phase V-I Measurement1/RConn1 -- Network equivalent/LConn1
  Network equivalent/RConn2 -- Network equivalent2/LConn2 -- Three-Phase Breaker2/LConn2
  Network equivalent/RConn3 -- Three-Phase Breaker2/LConn3 -- Network equivalent2/LConn3
  Network equivalent/RConn1 -- Three-Phase Breaker2/LConn1 -- Breaker/LConn1 -- Network equivalent2/LConn1
  Subsystem2/RConn4 -- Series RLC Branch/LConn1
  Series RLC Branch1/RConn1 -- Subsystem3/RConn4
  Series RLC Load/LConn1 -- Breaker/RConn1
  Series RLC Load3/LConn1 -- Three-Phase Breaker2/RConn2
  Series RLC Load2/LConn1 -- Three-Phase Breaker2/RConn1
  Series RLC Load4/LConn1 -- Three-Phase Breaker2/RConn3

== system PI_VC_vs_UPI_CC_3ph_4w_v2023b/Control PI_VC/PLL ==
  v_sabc : Inport
  Demux : Demux  Outputs=2
  Discrete-Time Integrator1 : DiscreteIntegrator  SampleTime=Ts_Control  ICPrevOutput=DiscIntNeverNeededParam  ICPrevScaledInput=DiscIntNeverNeededParam
  Integrator with Wrapped State (Discrete or Continuous) : eeGeneralControl/Integrator with Wrapped State (Discrete or Continuous)  LabelModeActiveChoice=Discrete  WrappedStateUpperValue=2*pi  WrappedStateLowerValue=0  x0=0  Ts=Ts_Control
  Ki : Gain  Gain=K_i_pll
  Kp : Gain  Gain=K_p_pll
  MATLAB Function1 : MATLAB Function  TreatAsAtomicUnit=on
  Sum : Sum  Inputs=|++
  omega : Outport  VectorParamsAs1DForOutWhenUnconnected=off
  theta : Outport  Port=2  VectorParamsAs1DForOutWhenUnconnected=off
  wires:
  MATLAB Function1/1(dq) -> Demux/1
  v_sabc/1 -> MATLAB Function1/2(abc)
  [theta] -> MATLAB Function1/1(theta)
  Ki/1 -> Discrete-Time Integrator1/1
  Kp/1 -> Sum/1
  Discrete-Time Integrator1/1 -> Sum/2
  Sum/1 -> Integrator with Wrapped State (Discrete or Continuous)/1, omega/1
  Integrator with Wrapped State (Discrete or Continuous)/1 -> [theta], theta/1
  Demux/1 -> Ki/1, Kp/1

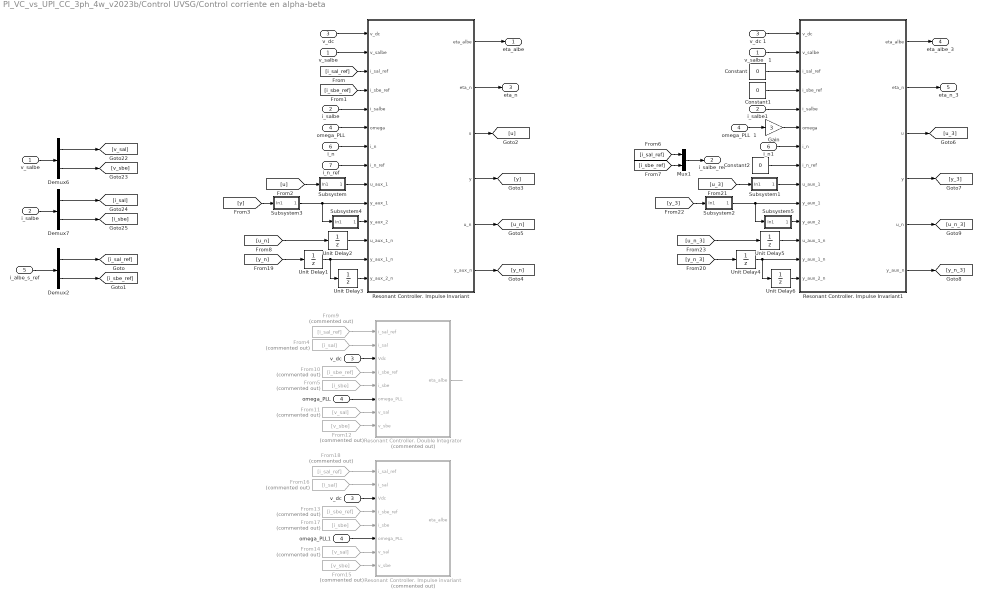
== system PI_VC_vs_UPI_CC_3ph_4w_v2023b/Control UVSG/Control corriente en alpha-beta ==
  v_salbe : Inport
  "i_salbe  " : Inport  Port=2
  v_dc : Inport  Port=3
  omega_PLL : Inport  Port=4
  i_albe_s_ref : Inport  Port=5
  i_n : Inport  Port=6
  i_n_ref : Inport  Port=7
  Constant : Constant  Value=0
  Constant1 : Constant  Value=0
  Constant2 : Constant  Value=0
  Demux2 : Demux  Outputs=2
  Demux6 : Demux  Outputs=2
  Demux7 : Demux  Outputs=2
  From10 : From  Commented=on  GotoTag=i_sbe_ref
  From11 : From  Commented=on  GotoTag=v_sal
  From12 : From  Commented=on  GotoTag=v_sbe
  From13 : From  Commented=on  GotoTag=i_sbe_ref
  From14 : From  Commented=on  GotoTag=v_sal
  From15 : From  Commented=on  GotoTag=v_sbe
  From16 : From  Commented=on  GotoTag=i_sal
  From17 : From  Commented=on  GotoTag=i_sbe
  From18 : From  Commented=on  GotoTag=i_sal_ref
  From4 : From  Commented=on  GotoTag=i_sal
  From5 : From  Commented=on  GotoTag=i_sbe
  From9 : From  Commented=on  GotoTag=i_sal_ref
  Gain : Gain  Gain=3
  Mux1 : Mux  Inputs=2
  Resonant Controller. Double Integrator : Subsystem  Commented=on
  Resonant Controller. Impulse Invariant : MATLAB Function  TreatAsAtomicUnit=on
  Resonant Controller. Impulse Invariant1 : MATLAB Function  TreatAsAtomicUnit=on
  Resonant Controller. Impulse invariant : Subsystem  Commented=on
  Subsystem : Subsystem
  Subsystem1 : Subsystem
  Subsystem2 : Subsystem
  Subsystem3 : Subsystem
  Subsystem4 : Subsystem
  Subsystem5 : Subsystem
  Unit Delay{1..6} (6 alike) : UnitDelay  SampleTime=Ts_Control  HasFrameUpgradeWarning=on
  i_n1 : InportShadow  Port=6
  i_salbe : InportShadow  Port=2
  i_salbe1 : InportShadow  Port=2
  "omega_PLL  " : InportShadow  Port=4
  omega_PLL  1 : InportShadow  Port=4
  omega_PLL1 : InportShadow  Port=4
  "v_dc " : InportShadow  Port=3
  "v_dc  " : InportShadow  Port=3
  v_dc 1 : InportShadow  Port=3
  "v_salbe   " : InportShadow
  v_salbe   1 : InportShadow
  eta_albe : Outport  VectorParamsAs1DForOutWhenUnconnected=off
  i_salbe_ref : Outport  Port=2  VectorParamsAs1DForOutWhenUnconnected=off
  eta_n : Outport  Port=3  VectorParamsAs1DForOutWhenUnconnected=off
  eta_albe_3 : Outport  Port=4  VectorParamsAs1DForOutWhenUnconnected=off
  eta_n_3 : Outport  Port=5  VectorParamsAs1DForOutWhenUnconnected=off
  wires:
  Demux6/1 -> [v_sal]
  Demux7/2 -> [i_sbe]
  Demux6/2 -> [v_sbe]
  Demux7/1 -> [i_sal]
  "i_salbe  "/1 -> Demux7/1
  v_salbe/1 -> Demux6/1
  Mux1/1 -> i_salbe_ref/1
  [i_sal_ref] -> Resonant Controller. Impulse Invariant/3(i_sal_ref)
  [i_sbe_ref] -> Resonant Controller. Impulse Invariant/4(i_sbe_ref)
  i_salbe/1 -> Resonant Controller. Impulse Invariant/5(i_salbe)
  "omega_PLL  "/1 -> Resonant Controller. Impulse Invariant/6(omega)
  Resonant Controller. Impulse Invariant/3(u) -> [u]
  Resonant Controller. Impulse Invariant/4(y) -> [y]
  [y] -> Subsystem3/1(In1)
  "v_salbe   "/1 -> Resonant Controller. Impulse Invariant/2(v_salbe)
  "v_dc "/1 -> Resonant Controller. Impulse Invariant/1(v_dc)
  Resonant Controller. Impulse Invariant/1(eta_albe) -> eta_albe/1
  [i_sal_ref] -> Mux1/1
  [i_sbe_ref] -> Mux1/2
  [u] -> Subsystem/1(In1)
  Subsystem/1(Out1) -> Resonant Controller. Impulse Invariant/9(u_aux_1)
  Subsystem4/1(Out1) -> Resonant Controller. Impulse Invariant/11(y_aux_2)
  Subsystem3/1(Out1) -> Resonant Controller. Impulse Invariant/10(y_aux_1), Subsystem4/1(In1)
  From9/1 -> Resonant Controller. Double Integrator/1(i_sal_ref)
  From4/1 -> Resonant Controller. Double Integrator/2(i_sal)
  v_dc/1 -> Resonant Controller. Double Integrator/3(Vdc)
  From10/1 -> Resonant Controller. Double Integrator/4(i_sbe_ref)
  From5/1 -> Resonant Controller. Double Integrator/5(i_sbe)
  omega_PLL/1 -> Resonant Controller. Double Integrator/6(omega_PLL)
  Resonant Controller. Double Integrator/1(eta_albe) -> ?
  From11/1 -> Resonant Controller. Double Integrator/7(v_sal)
  From12/1 -> Resonant Controller. Double Integrator/8(v_sbe)
  From14/1 -> Resonant Controller. Impulse invariant/7(v_sal)
  omega_PLL1/1 -> Resonant Controller. Impulse invariant/6(omega_PLL)
  From17/1 -> Resonant Controller. Impulse invariant/5(i_sbe)
  From16/1 -> Resonant Controller. Impulse invariant/2(i_sal)
  "v_dc  "/1 -> Resonant Controller. Impulse invariant/3(Vdc)
  From13/1 -> Resonant Controller. Impulse invariant/4(i_sbe_ref)
  From18/1 -> Resonant Controller. Impulse invariant/1(i_sal_ref)
  From15/1 -> Resonant Controller. Impulse invariant/8(v_sbe)
  i_albe_s_ref/1 -> Demux2/1
  Demux2/1 -> [i_sal_ref]
  Demux2/2 -> [i_sbe_ref]
  i_n/1 -> Resonant Controller. Impulse Invariant/7(i_n)
  i_n_ref/1 -> Resonant Controller. Impulse Invariant/8(i_n_ref)
  Resonant Controller. Impulse Invariant/2(eta_n) -> eta_n/1
  Resonant Controller. Impulse Invariant/6(y_aux_n) -> [y_n]
  Resonant Controller. Impulse Invariant/5(u_n) -> [u_n]
  Unit Delay2/1 -> Resonant Controller. Impulse Invariant/12(u_aux_1_n)
  [u_n] -> Unit Delay2/1
  [y_n] -> Unit Delay1/1
  Unit Delay1/1 -> Resonant Controller. Impulse Invariant/13(y_aux_1_n), Unit Delay3/1
  Unit Delay3/1 -> Resonant Controller. Impulse Invariant/14(y_aux_2_n)
  v_dc 1/1 -> Resonant Controller. Impulse Invariant1/1(v_dc)
  v_salbe   1/1 -> Resonant Controller. Impulse Invariant1/2(v_salbe)
  Constant/1 -> Resonant Controller. Impulse Invariant1/3(i_sal_ref)
  Constant1/1 -> Resonant Controller. Impulse Invariant1/4(i_sbe_ref)
  i_salbe1/1 -> Resonant Controller. Impulse Invariant1/5(i_salbe)
  omega_PLL  1/1 -> Gain/1
  Gain/1 -> Resonant Controller. Impulse Invariant1/6(omega)
  i_n1/1 -> Resonant Controller. Impulse Invariant1/7(i_n)
  Constant2/1 -> Resonant Controller. Impulse Invariant1/8(i_n_ref)
  Unit Delay4/1 -> Resonant Controller. Impulse Invariant1/13(y_aux_1_n), Unit Delay6/1
  [y_n_3] -> Unit Delay4/1
  [u_n_3] -> Unit Delay5/1
  Subsystem2/1(Out1) -> Resonant Controller. Impulse Invariant1/10(y_aux_1), Subsystem5/1(In1)
  [u_3] -> Subsystem1/1(In1)
  [y_3] -> Subsystem2/1(In1)
  Subsystem1/1(u_aux_1) -> Resonant Controller. Impulse Invariant1/9(u_aux_1)
  Unit Delay5/1 -> Resonant Controller. Impulse Invariant1/12(u_aux_1_n)
  Unit Delay6/1 -> Resonant Controller. Impulse Invariant1/14(y_aux_2_n)
  Resonant Controller. Impulse Invariant1/1(eta_albe) -> eta_albe_3/1
  Resonant Controller. Impulse Invariant1/2(eta_n) -> eta_n_3/1
  Resonant Controller. Impulse Invariant1/3(u) -> [u_3]
  Resonant Controller. Impulse Invariant1/4(y) -> [y_3]
  Resonant Controller. Impulse Invariant1/5(u_n) -> [u_n_3]
  Resonant Controller. Impulse Invariant1/6(y_aux_n) -> [y_n_3]
  Subsystem5/1(y_aux_2) -> Resonant Controller. Impulse Invariant1/11(y_aux_2)

== system PI_VC_vs_UPI_CC_3ph_4w_v2023b/Control UVSG/PARK_PLL ==
  note: PLL US
  v_sabc : Inport
  eta_albe : Inport  Port=2
  i_sabc : Inport  Port=3
  i_abc_s_ref : Inport  Port=4
  Constant{1..4} (4 alike) : Constant  Value=0
  MATLAB Function1 : MATLAB Function  TreatAsAtomicUnit=on
  MATLAB Function2 : MATLAB Function  TreatAsAtomicUnit=on
  MATLAB Function3 : MATLAB Function  TreatAsAtomicUnit=on
  MATLAB Function5 : MATLAB Function  TreatAsAtomicUnit=on
  PLL : Subsystem
  "v_sabc " : InportShadow
  v_salbe : Outport  VectorParamsAs1DForOutWhenUnconnected=off
  eta_abc : Outport  Port=2  VectorParamsAs1DForOutWhenUnconnected=off
  theta : Outport  Port=3  VectorParamsAs1DForOutWhenUnconnected=off
  i_salbe : Outport  Port=4  VectorParamsAs1DForOutWhenUnconnected=off
  omega : Outport  Port=5  VectorParamsAs1DForOutWhenUnconnected=off
  i_albe_s_ref : Outport  Port=6  VectorParamsAs1DForOutWhenUnconnected=off
  wires:
  Constant1/1 -> MATLAB Function3/1(theta)
  v_sabc/1 -> MATLAB Function3/2(abc)
  MATLAB Function3/1(dq) -> v_salbe/1
  Constant2/1 -> MATLAB Function1/1(theta)
  i_sabc/1 -> MATLAB Function1/2(abc)
  MATLAB Function1/1(dq) -> i_salbe/1
  eta_albe/1 -> MATLAB Function5/2(dq)
  Constant3/1 -> MATLAB Function5/1(theta)
  MATLAB Function5/1(abc) -> eta_abc/1
  PLL/2(theta) -> theta/1
  PLL/1(omega) -> omega/1
  "v_sabc "/1 -> PLL/1(v_sabc)
  i_abc_s_ref/1 -> MATLAB Function2/2(abc)
  Constant4/1 -> MATLAB Function2/1(theta)
  MATLAB Function2/1(dq) -> i_albe_s_ref/1
